simulink model "exOne"  (R2014a)
settings: Solver=ode45  StartTime=0.0  StopTime=10.0  RelTol=1e-3
values from neighbouring files (symbols this model uses):
  d = 10    [bookEx.m]    (also in massSpring.m = 5)
  F = A1-K1*C    [bookEx.m]    (also in carsus.m = diag(v); massSpring.m)
  K = K1 + F*H    [bookEx.m]    (also in massSpring.m)
  x1_0 = 100    [bookEx.m]    (also in massSpring.m = -1)
  x2_0 = -100    [bookEx.m]    (also in massSpring.m = -5)
  x3_0 = 1    [bookEx.m]    (also in massSpring.m)
settings Model: Creator=sqn4594  LastModifiedBy=sqn4594

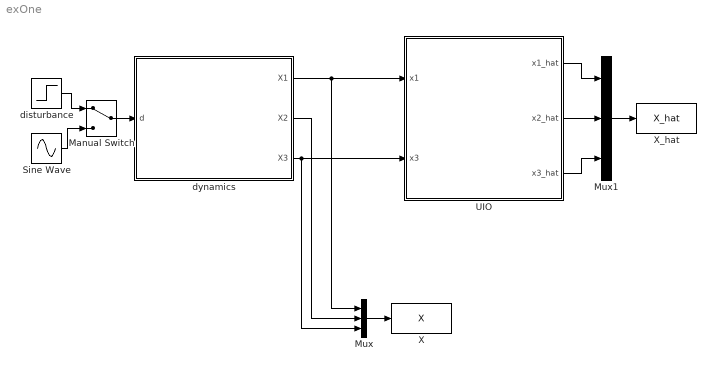
== system exOne ==
  Manual Switch : ManualSwitch
  Mux : Mux  Inputs=3
  Mux1 : Mux  Inputs=3
  Sine Wave : Sin  Amplitude=20  Frequency=2  SampleTime=0
  UIO : Subsystem
  X : ToWorkspace  VariableName=X  SampleTime=-1
  X_hat : ToWorkspace  VariableName=X_hat  SampleTime=-1
  disturbance : Step  After=d  SampleTime=0
  dynamics : Subsystem
  wires:
  dynamics/3(X3) -> Mux/3, UIO/2(x3)
  dynamics/1(X1) -> Mux/1, UIO/1(x1)
  Mux/1 -> X/1
  dynamics/2(X2) -> Mux/2
  UIO/2(x2_hat) -> Mux1/2
  UIO/3(x3_hat) -> Mux1/3
  UIO/1(x1_hat) -> Mux1/1
  Mux1/1 -> X_hat/1
  Manual Switch/1 -> dynamics/1(d)
  disturbance/1 -> Manual Switch/1
  Sine Wave/1 -> Manual Switch/2

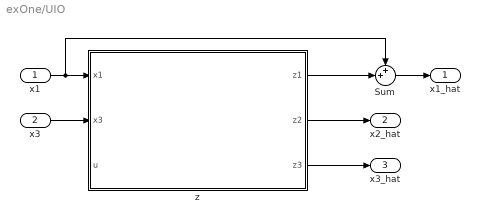
== system exOne/UIO ==
  x1 : Inport
  x3 : Inport  Port=2
  Sum : Sum  Inputs=++|
  z : Subsystem
  x1_hat : Outport
  x2_hat : Outport  Port=2
  x3_hat : Outport  Port=3
  wires:
  x1/1 -> Sum/1, z/1(x1)
  x3/1 -> z/2(x3)
  z/1(z1) -> Sum/2
  Sum/1 -> x1_hat/1
  z/2(z2) -> x2_hat/1
  z/3(z3) -> x3_hat/1

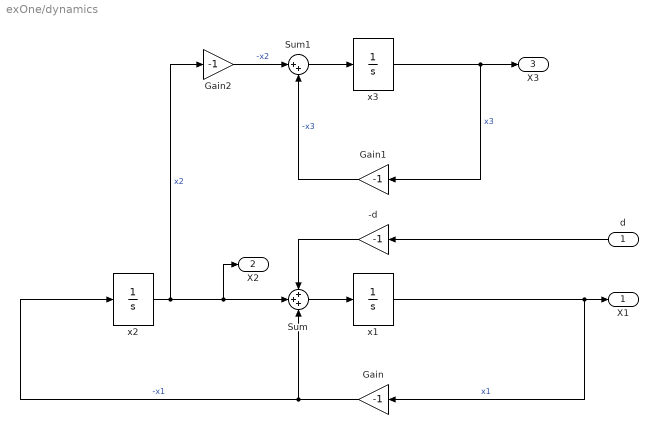
== system exOne/dynamics ==
  d : Inport
  -d : Gain  Gain=-1
  Gain : Gain  Gain=-1
  Gain1 : Gain  Gain=-1
  Gain2 : Gain  Gain=-1
  Sum : Sum  Inputs=+++
  Sum1 : Sum  Inputs=|++
  x1 : Integrator  InitialCondition=x1_0
  x2 : Integrator  InitialCondition=x2_0
  x3 : Integrator  InitialCondition=x3_0
  X1 : Outport
  X2 : Outport  Port=2
  X3 : Outport  Port=3
  wires:
  x1/1 -> X1/1, Gain/1  "x1"
  x2/1 -> Gain2/1, Sum/2, X2/1  "x2"
  Gain2/1 -> Sum1/1  "-x2"
  Gain/1 -> Sum/3, x2/1  "-x1"
  Sum/1 -> x1/1
  x3/1 -> X3/1, Gain1/1  "x3"
  Sum1/1 -> x3/1
  Gain1/1 -> Sum1/2  "-x3"
  d/1 -> -d/1
  -d/1 -> Sum/1

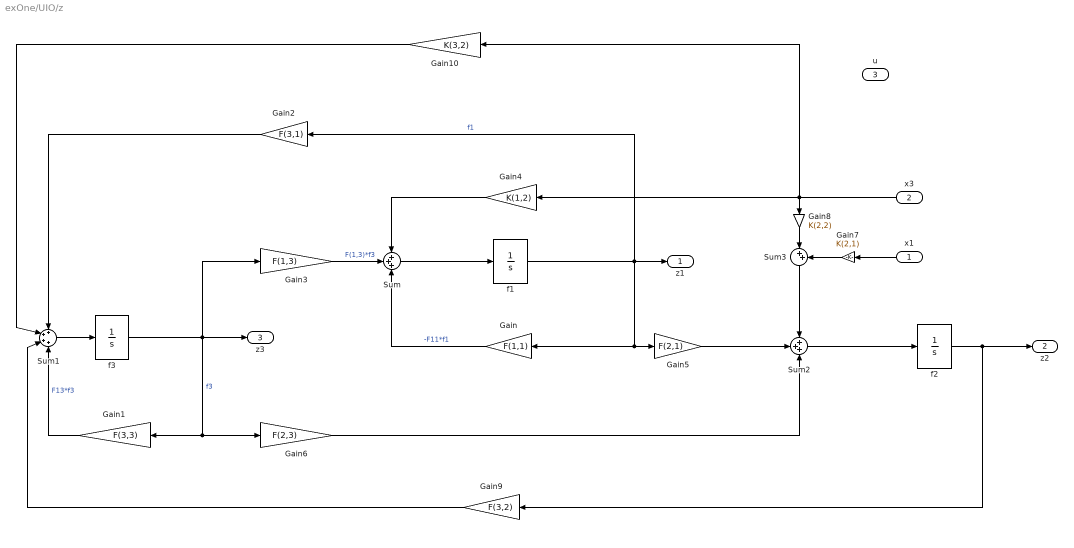
== system exOne/UIO/z ==
  x1 : Inport
  x3 : Inport  Port=2
  u : Inport  Port=3
  Gain : Gain  Gain=F(1,1)
  Gain1 : Gain  Gain=F(3,3)
  Gain10 : Gain  Gain=K(3,2)
  Gain2 : Gain  Gain=F(3,1)
  Gain3 : Gain  Gain=F(1,3)
  Gain4 : Gain  Gain=K(1,2)
  Gain5 : Gain  Gain=F(2,1)
  Gain6 : Gain  Gain=F(2,3)
  Gain7 : Gain  Gain=K(2,1)
  Gain8 : Gain  Gain=K(2,2)
  Gain9 : Gain  Gain=F(3,2)
  Sum : Sum  Inputs=+++
  Sum1 : Sum  Inputs=++++
  Sum2 : Sum  Inputs=+++
  Sum3 : Sum  Inputs=|++
  f1 : Integrator  InitialCondition=x1_0
  f2 : Integrator  InitialCondition=x1_0
  f3 : Integrator  InitialCondition=x3_0
  z1 : Outport
  z2 : Outport  Port=2
  z3 : Outport  Port=3
  wires:
  Sum2/1 -> f2/1
  Sum3/1 -> Sum2/1
  f2/1 -> z2/1, Gain9/1
  x3/1 -> Gain10/1, Gain8/1, Gain4/1
  Gain10/1 -> Sum1/2
  Gain9/1 -> Sum1/3
  Gain2/1 -> Sum1/1
  Gain/1 -> Sum/3  "-F11*f1"
  Gain6/1 -> Sum2/3
  Gain5/1 -> Sum2/2
  Gain4/1 -> Sum/1
  Gain7/1 -> Sum3/2
  x1/1 -> Gain7/1
  Gain3/1 -> Sum/2  "F(1,3)*f3"
  Gain8/1 -> Sum3/1
  Sum/1 -> f1/1
  f1/1 -> z1/1, Gain5/1, Gain/1, Gain2/1  "f1"
  Gain1/1 -> Sum1/4  "F13*f3"
  Sum1/1 -> f3/1
  f3/1 -> z3/1, Gain3/1, Gain1/1, Gain6/1  "f3"
